simulink model "dr"  (R2025b)
settings: Solver=ode45  StartTime=0.0  StopTime=10000  RelTol=1e-6  AbsTol=1e-6
settings Model: Creator=arxchy  LastModifiedBy=arxchy

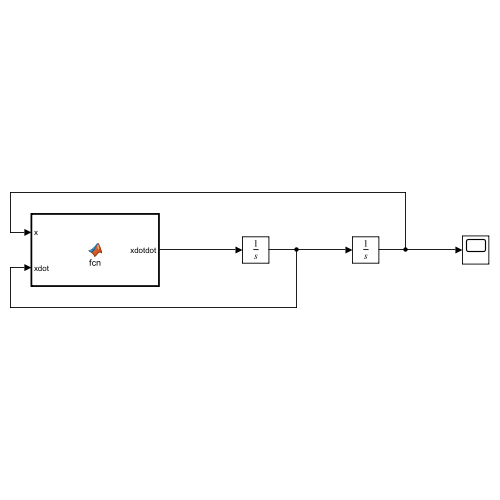
[thumbnail: Simulink's stored preview of the top-level diagram]
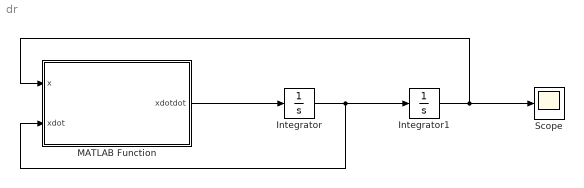
== system dr ==
  Integrator : Integrator
  Integrator1 : Integrator  InitialCondition=1
  MATLAB Function : MATLAB Function  TreatAsAtomicUnit=on
  Scope : Scope
      settings: ActiveDisplayYMinimum=-0.15756141358949216  ActiveDisplayYMaximum=0.39051550600687945
  wires:
  Integrator1/1 -> MATLAB Function/1(x), Scope/1
  Integrator/1 -> MATLAB Function/2(xdot), Integrator1/1
  MATLAB Function/1(xdotdot) -> Integrator/1

== matlab function dr/MATLAB Function ==
  data: x input; xdot input; xdotdot output
function xdotdot = fcn(x, xdot)

xdotdot = -0.1*xdot - 10*x;
